simulink model "IC125_K2K_FCB"  (R2018a)
settings: Solver=ode23tb  StartTime=0.0  StopTime=inf  EnableMultiTasking=on
InitFcn:
  | clc
  | init
values from neighbouring files (symbols this model uses):
  C = ( Vout * ( 1 - D ) )/ ( 8 * L * fs^2 * delta_Vout )    (= 0.00125)    [init.m]
  Davis = [6 0.21 0.01453 0].*(404/752.4)    [vehicle_IC125.m]
  gradient_prof_interp_spline_matrix = [0 0.01 0.02 0.03 0.04 0.05 0.06 0.07 0.08 0.09 0.1 0.11 ... (345742 elements, 172871x2)]    [gradient_prof_interp_spline_matrix_kx.mat]    (also in two_way_gradient_interpolated.mat = [1 1.01 1.02 1.03 1.04 1.05 1.06 1.07 1.08 1.09 1.1 1.11 ...)
  inertial_mass = Mass*(1+lambda)    [vehicle_IC125.m]
  L = ( Vout * ( Vin - Vout ) ) / ( Vin * fs * delta_iL )    (= 3.75)    [init.m]
  L_boost = ( Vin_boost * ( Vout_boost - Vin_boost ) ) / ( Vout_boost * delta_iL * fs_boost )    (= 0.0586666666667)    [init.m]
  lambda = 0.08    [vehicle_IC125.m]
  radius = 0.4064    [init.m]
  vel_profile = [0 0.43434 0.4425696 0.4489704 0.4553712 0.461772 0.603504 0.9153144 0.9253728 0.928116 1.0296144 1.0314432 ... (6854 elements, 3427x2)]    [route_KingsX_NewC_KingsX.mat]
undefined symbols (not defined in the file or in its folder): gradient_prof, Ion, Lithium
libraries: powerlib x30, simulink x9, powerlib_meascontrol x5, electricdrivelib x2
settings Model: Creator=hegazi  LastModifiedBy=hegazi
settings SolverCC: ZeroCrossControl=DisableAll  DecoupledContinuousIntegration=on
settings DataIOCC: SaveFormat=Structure  SaveOutput=off  SaveState=on  SignalLogging=off  DSMLogging=off  ReturnWorkspaceOutputs=on  ReturnWorkspaceOutputsName=tp19da9ac7_18bf_45fb_8707_61b44884cc90
settings OptimizationCC: EfficientMapNaN2IntZero=off  LifeSpan=inf
settings DebuggingCC: SFUnexpectedBacktrackingDiag=warning  SFNoUnconditionalDefaultTransitionDiag=warning  SFExecutionAtInitializationDiag=none
settings HardwareCC: ProdBitPerPointer=32  ProdBitPerSizeT=32  ProdBitPerPtrDiffT=32  ProdLargestAtomicFloat=None  ProdIntDivRoundTo=Undefined  ProdEndianess=Unspecified  ProdWordSize=32  ProdHWDeviceType=32-bit Generic  TargetBitPerPointer=64  TargetBitPerSizeT=64  TargetBitPerPtrDiffT=64  TargetLongLongMode=on  TargetIntDivRoundTo=Zero  TargetEndianess=LittleEndian  TargetWordSize=64  TargetHWDeviceType=MATLAB Host  ProdEqTarget=off
settings ModelReferenceCC: PropagateSignalLabelsOutOfModel=off
settings CodeAppCC: MaxIdLength=128
settings GRTTargetCC: TargetLangStandard=C89/C90 (ANSI)  CombineOutputUpdateFcns=off  GRTInterface=on
settings ConfigComp: CovMetricSettings=dw  CovHtmlReporting=on  CovSaveCumulativeToWorkspaceVar=on  CovSaveSingleToWorkspaceVar=on  CovExternalEMLEnable=off
settings SimscapeCC: SimscapeNormalizeSystem=off  SimscapeLogType=all  SimscapeLogSimulationStatistics=on  SimscapeLogLimitData=off

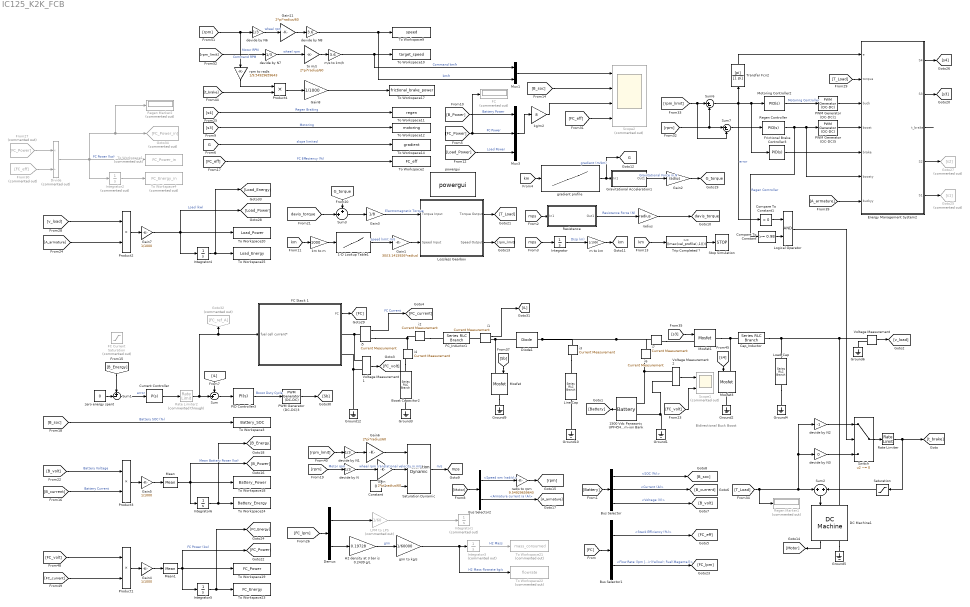
== system IC125_K2K_FCB ==
  note: Bidirectional Buck Boost
  1-D Lookup Table1 : Lookup_n-D  NumberOfTableDimensions=1  BreakpointsForDimension1=vel_profile(:,1)*1000  BreakpointsForDimension2=linspace(min(gradient_prof(:,2)),max(gradient_prof(:,2)),190)  BreakpointsForDimension1DataTypeStr=Inherit: Inherit from 'Breakpoint data'  IndexSearchMethod=Linear search  BeginIndexSearchUsingPreviousIndexResult=on  Table=vel_profile(:,2)*0.277778  TableDataTypeStr=Inherit: Inherit from 'Table data'  InterpMethod=Flat  RemoveProtectionInput=on  InternalRulePriority=Speed  RndMeth=Simplest  SaturateOnIntegerOverflow=on  InputSameDT=on
  1500 Vdc Panasonic UPF454261 Lithium-ion Bank : electricdrivelib/Extra Sources/Battery  BatType=Lithium-Ion  ShowTempParam=off  ThermalPreset=no  ShowAgeParam=off  NomV=3.7*405  NomQ=50  SOC=50  Batt_Tr=30  PresetModel=on  MaxQ=50  MinV=1123.875  FullV=1744.2347  Dis_rate=21.7391  R=0.2997  Normal_OP=45.2174  expZone="[1618.9582      2.4565217]"  current=[1.5 3]  Units=Ampere-hour  Tci=20  NomT=25  T2=0  MaxQ2=2.208  FullV2=3.45  Normal_OP2=2.8  expZone2="[3.22        0.23]"  Rca=0.6  ti=1000  Dp=0  Neq0=0  Tsim=1e6  Ta1=25  Qeol=5.4*0.9  Reol=0.013333*1.2  Char_age=[2.3478, 3]  Dis_age=[2.3478, 10]  N1=1500  N2=10500  N3=1000  N4=1400  Ta2=45  N5=950
  Boost Capacitor2 : powerlib/Elements/Series RLC Branch  LConnTagsString=__new0  RConnTagsString=__new0  BranchType=RC  Resistance=1  Inductance=1e-3  SetiL0=off  InitialCurrent=0  Capacitance=1e-3  Setx0=on  InitialVoltage=400  Measurements=None
  Bus Selector : BusSelector  OutputSignals=SOC (%),Current (A),Voltage (V)
  Bus Selector1 : BusSelector  OutputSignals=Stack Efficiency (%),Flow Rate (lpm [Air(Yellow); Fuel(Magenta)]
  Bus Selector2 : BusSelector  OutputSignals=Speed wm (rad/s),Armature current ia (A)
  Cap_Inductor : powerlib/Elements/Series RLC Branch  LConnTagsString=__new0  RConnTagsString=__new0  BranchType=L  Resistance=1  Inductance=L  SetiL0=off  InitialCurrent=1  Capacitance=1e-6  Setx0=off  InitialVoltage=0  Measurements=Branch voltage and current
  Compare To Constant : simulink/Logic and Bit Operations/Compare To Constant  relop=>=  const=0.98  OutDataTypeStr=boolean
  Compare To Constant1 : simulink/Logic and Bit Operations/Compare To Constant  relop=<  const=0  OutDataTypeStr=boolean
  Constant : Constant  Value=0
  Current Controller : simulink/Continuous/PID Controller  Controller=P  TimeDomain=Continuous-time  SampleTime=-1  IntegratorMethod=Forward Euler  FilterMethod=Forward Euler  Form=Parallel  UseFilter=on  ControllerParametersSource=internal  P=0.5  I=0.001  D=-6.1007201679259e-06  N=246.043739643854  InitialConditionSource=internal  InitialConditionForIntegrator=0  InitialConditionForFilter=0  ExternalReset=none  ZeroCross=off  LimitOutput=off  UpperSaturationLimit=300  LowerSaturationLimit=0  LinearizeAsGain=on  AntiWindupMode=none  Kb=1  TrackingMode=off  Kt=1  PParamMin=[]  PParamMax=[]  IParamMin=[]  IParamMax=[]  DParamMin=[]  DParamMax=[]  NParamMin=[]  NParamMax=[]  KbParamMin=[]  KbParamMax=[]  KtParamMin=[]  KtParamMax=[]  POutMin=[]  POutMax=[]  IOutMin=[]  IOutMax=[]  DOutMin=[]  DOutMax=[]  NOutMin=[]  NOutMax=[]  KbOutMin=[]  KbOutMax=[]  KtOutMin=[]  KtOutMax=[]  IntegratorOutMin=[]  IntegratorOutMax=[]  FilterOutMin=[]  FilterOutMax=[]  SumOutMin=[]  SumOutMax=[]  SumI1OutMin=[]  SumI1OutMax=[]  SumI2OutMin=[]  SumI2OutMax=[]  SumI3OutMin=[]  SumI3OutMax=[]  SumDOutMin=[]  SumDOutMax=[]  SaturationOutMin=[]  SaturationOutMax=[]  IntegratorContinuousStateAttributes=''  IntegratorStateMustResolveToSignalObject=off  IntegratorRTWStateStorageClass=Auto  FilterContinuousStateAttributes=''  FilterStateMustResolveToSignalObject=off  FilterRTWStateStorageClass=Auto  DifferentiatorICPrevScaledInput=0  DifferentiatorOutMin=[]  DifferentiatorOutMax=[]  InitialConditionSetting=State (most efficient)  FilterDiffOutCoefMin=[]  FilterDiffOutCoefMax=[]  SumDenOutMin=[]  SumDenOutMax=[]  SumNumOutMin=[]  SumNumOutMax=[]  ReciprocalOutMin=[]  ReciprocalOutMax=[]  DivideOutMin=[]  DivideOutMax=[]  TunerSelectOption=Transfer Function Based (PID Tuner App)
  DC Machine1 : powerlib/Machines/DC Machine  PresetModel=No  MechanicalLoad=Torque TL  FieldType=Permanent magnet  ShowDetailedParameters=on  MeasurementBus=off  RLa=[0.1499 0.002884]  RLf=[51.14 5.968]  Laf=0.4365  MachineConstant=Torque constant (N.m/A)  Ke=1.8  Kt=1.8  J=0.5106  Bm=0.01383  Tf=13.22  w0=1*(vel_profile(1,2)./(2*pi*radius/60)*3)/9.54929659643  Ifinit=0  TsPowergui=0  TsBlock=-1
  Demux : Demux  Outputs=2
  Diode1 : powerlib/Power Electronics/Diode  Ron=0.001  Lon=0  Vf=0.8  IC=0  UseSnubber=off  Rs=500  Cs=250e-9  Measurements=off
  Divide : Product  Commented=on  Inputs=*/
  Energy Management System2 : State Transition Table  TreatAsAtomicUnit=on
  FC : Display  Commented=on
  FC Current Saturation : Saturate  Commented=on  UpperLimit=50  LowerLimit=0  OutMax=62.5
  FC Stack 1 : Subsystem
      mask Display: image(imread('power_FCV_powertrain_stack.bmp'))
  FC_Inductor1 : powerlib/Elements/Series RLC Branch  LConnTagsString=__new0  RConnTagsString=__new0  BranchType=L  Resistance=0.1  Inductance=L_boost  SetiL0=off  InitialCurrent=1  Capacitance=1e-6  Setx0=off  InitialVoltage=0  Measurements=Branch voltage and current
  Frictional Brake Controller3 : simulink/Continuous/PID Controller  Controller=PID  TimeDomain=Continuous-time  SampleTime=-1  IntegratorMethod=Forward Euler  FilterMethod=Forward Euler  Form=Parallel  UseFilter=on  ControllerParametersSource=internal  P=-0.214642815578935  I=-0.15951379317719  D=-0.00934490052913337  N=15.3222973940802  InitialConditionSource=internal  InitialConditionForIntegrator=0  InitialConditionForFilter=0  ExternalReset=none  LimitOutput=off  UpperSaturationLimit=inf  LowerSaturationLimit=0  LinearizeAsGain=on  AntiWindupMode=none  Kb=1  TrackingMode=off  Kt=1  PParamMin=[]  PParamMax=[]  IParamMin=[]  IParamMax=[]  DParamMin=[]  DParamMax=[]  NParamMin=[]  NParamMax=[]  KbParamMin=[]  KbParamMax=[]  KtParamMin=[]  KtParamMax=[]  POutMin=[]  POutMax=[]  IOutMin=[]  IOutMax=[]  DOutMin=[]  DOutMax=[]  NOutMin=[]  NOutMax=[]  KbOutMin=[]  KbOutMax=[]  KtOutMin=[]  KtOutMax=[]  IntegratorOutMin=[]  IntegratorOutMax=[]  FilterOutMin=[]  FilterOutMax=[]  SumOutMin=[]  SumOutMax=[]  SumI1OutMin=[]  SumI1OutMax=[]  SumI2OutMin=[]  SumI2OutMax=[]  SumI3OutMin=[]  SumI3OutMax=[]  SumDOutMin=[]  SumDOutMax=[]  SaturationOutMin=[]  SaturationOutMax=[]  IntegratorContinuousStateAttributes=''  IntegratorStateMustResolveToSignalObject=off  IntegratorRTWStateStorageClass=Auto  FilterContinuousStateAttributes=''  FilterStateMustResolveToSignalObject=off  FilterRTWStateStorageClass=Auto  DifferentiatorICPrevScaledInput=0  DifferentiatorOutMin=[]  DifferentiatorOutMax=[]  InitialConditionSetting=State (most efficient)  FilterDiffOutCoefMin=[]  FilterDiffOutCoefMax=[]  SumDenOutMin=[]  SumDenOutMax=[]  SumNumOutMin=[]  SumNumOutMax=[]  ReciprocalOutMin=[]  ReciprocalOutMax=[]  DivideOutMin=[]  DivideOutMax=[]  TunerSelectOption=Transfer Function Based (PID Tuner App)
  From27 : From  Commented=on  GotoTag=FC_Power
  From30 : From  Commented=on  GotoTag=FC_eff
  Gain : Gain  Gain=2*pi*radius/60
  Gain1 : Gain  Gain=30/(3.1415926*radius)
  Gain11 : Gain  Gain=2*pi*radius/60
  Gain2 : Gain  Gain=radius
  Gain3 : Gain  Gain=1/8
  Gain{4..5,7..8} (4 alike) : Gain  Gain=1/1000
  Gain6 : Gain  Gain=2*pi*radius/60
  Goto25 : Goto  Commented=on  GotoTag=s1
  Goto27 : Goto  Commented=on  GotoTag=s2
  Goto32 : Goto  Commented=on  GotoTag=FC_ref_A
  Goto34 : Goto  Commented=on  GotoTag=FC_Power_in
  Gravitational Acceleration1 : Subsystem
  Ground{1..6,9..10,12} (9 alike) : powerlib/Elements/Ground  LConnTagsString=a
  H2 density at 3 bar is 0.2439 g/L : Gain  Gain=0.19728
  Integrator : Integrator  InitialCondition=vel_profile(2,1)  ZeroCross=off
  Integrator1 : Integrator  Commented=on  ZeroCross=off
  Integrator2 : Integrator  Commented=on  LimitOutput=on  UpperSaturationLimit=500  LowerSaturationLimit=0  ZeroCross=off
  Integrator3 : Integrator  Commented=on  ZeroCross=off
  Integrator4 : Integrator  ZeroCross=off
  Integrator5 : Integrator  ZeroCross=off
  Integrator6 : Integrator  ZeroCross=off
  LPM to LPS : Gain  Commented=on  Gain=1/60
  Line Cap : powerlib/Elements/Series RLC Branch  LConnTagsString=__new0  RConnTagsString=__new0  BranchType=RC  Resistance=0.0000000000001  Inductance=1e-3  SetiL0=off  InitialCurrent=0  Capacitance=1e-1  Setx0=on  InitialVoltage=1580  Measurements=None
  Load_Cap : powerlib/Elements/Series RLC Branch  LConnTagsString=__new0  RConnTagsString=__new0  BranchType=C  Resistance=1  Inductance=1e-3  SetiL0=off  InitialCurrent=0  Capacitance=C*10  Setx0=off  InitialVoltage=500  Measurements=Branch voltage and current
  Logical Operator : Logic  AllPortsSameDT=off  OutDataTypeStr=boolean
  Lossless Gearbox : Subsystem  mask{N=3}
      mask prompts: N "Gear Ratio"
      mask Display: image(imread('gearbox.jpg'))
  Mean : powerlib_meascontrol/Measurements/Mean  Freq=1  Vinit=0  Ts=0
  Mean1 : powerlib_meascontrol/Measurements/Mean  Freq=1  Vinit=0  Ts=0
  Mosfet : powerlib/Power Electronics/Mosfet  Ron=0.1  Lon=0  Rd=0.01  Vfd=0  IC=0  Rs=1e5  Cs=inf  Measurements=off
  Mosfet1 : powerlib/Power Electronics/Mosfet  Ron=0.1  Lon=0  Rd=0.01  Vfd=0  IC=0  Rs=1e5  Cs=inf  Measurements=off
  Mosfet3 : powerlib/Power Electronics/Mosfet  Ron=0.1  Lon=0  Rd=0.01  Vfd=0  IC=0  Rs=1e5  Cs=inf  Measurements=off
  Motoring Controller2 : simulink/Continuous/PID Controller  Controller=PID  TimeDomain=Continuous-time  SampleTime=-1  IntegratorMethod=Forward Euler  FilterMethod=Forward Euler  Form=Parallel  UseFilter=on  ControllerParametersSource=internal  P=0.0168081368407346  I=0.01166650788265202  D=0.00626354102809722  N=66.8094473612698  InitialConditionSource=internal  InitialConditionForIntegrator=0  InitialConditionForFilter=0  ExternalReset=none  ZeroCross=off  LimitOutput=on  UpperSaturationLimit=1  LowerSaturationLimit=0  LinearizeAsGain=on  AntiWindupMode=none  Kb=1  TrackingMode=off  Kt=1  PParamMin=[]  PParamMax=[]  IParamMin=[]  IParamMax=[]  DParamMin=[]  DParamMax=[]  NParamMin=[]  NParamMax=[]  KbParamMin=[]  KbParamMax=[]  KtParamMin=[]  KtParamMax=[]  POutMin=[]  POutMax=[]  IOutMin=[]  IOutMax=[]  DOutMin=[]  DOutMax=[]  NOutMin=[]  NOutMax=[]  KbOutMin=[]  KbOutMax=[]  KtOutMin=[]  KtOutMax=[]  IntegratorOutMin=[]  IntegratorOutMax=[]  FilterOutMin=[]  FilterOutMax=[]  SumOutMin=[]  SumOutMax=[]  SumI1OutMin=[]  SumI1OutMax=[]  SumI2OutMin=[]  SumI2OutMax=[]  SumI3OutMin=[]  SumI3OutMax=[]  SumDOutMin=[]  SumDOutMax=[]  SaturationOutMin=[]  SaturationOutMax=[]  IntegratorContinuousStateAttributes=''  IntegratorStateMustResolveToSignalObject=off  IntegratorRTWStateStorageClass=Auto  FilterContinuousStateAttributes=''  FilterStateMustResolveToSignalObject=off  FilterRTWStateStorageClass=Auto  DifferentiatorICPrevScaledInput=0  DifferentiatorOutMin=[]  DifferentiatorOutMax=[]  InitialConditionSetting=State (most efficient)  FilterDiffOutCoefMin=[]  FilterDiffOutCoefMax=[]  SumDenOutMin=[]  SumDenOutMax=[]  SumNumOutMin=[]  SumNumOutMax=[]  ReciprocalOutMin=[]  ReciprocalOutMax=[]  DivideOutMin=[]  DivideOutMax=[]  TunerSelectOption=Transfer Function Based (PID Tuner App)
  Mux1 : Mux  Inputs=2
  Mux3 : Mux  Inputs=3
  PID Controller3 : simulink/Continuous/PID Controller  Controller=PI  TimeDomain=Continuous-time  SampleTime=-1  IntegratorMethod=Forward Euler  FilterMethod=Forward Euler  Form=Parallel  UseFilter=on  ControllerParametersSource=internal  P=0.00150104400463717  I=0.095515581062299  D=-6.1007201679259e-06  N=246.043739643854  InitialConditionSource=internal  InitialConditionForIntegrator=0  InitialConditionForFilter=0  ExternalReset=none  ZeroCross=off  LimitOutput=on  UpperSaturationLimit=1  LowerSaturationLimit=0  LinearizeAsGain=on  AntiWindupMode=none  Kb=1  TrackingMode=off  Kt=1  PParamMin=[]  PParamMax=[]  IParamMin=[]  IParamMax=[]  DParamMin=[]  DParamMax=[]  NParamMin=[]  NParamMax=[]  KbParamMin=[]  KbParamMax=[]  KtParamMin=[]  KtParamMax=[]  POutMin=[]  POutMax=[]  IOutMin=[]  IOutMax=[]  DOutMin=[]  DOutMax=[]  NOutMin=[]  NOutMax=[]  KbOutMin=[]  KbOutMax=[]  KtOutMin=[]  KtOutMax=[]  IntegratorOutMin=[]  IntegratorOutMax=[]  FilterOutMin=[]  FilterOutMax=[]  SumOutMin=[]  SumOutMax=[]  SumI1OutMin=[]  SumI1OutMax=[]  SumI2OutMin=[]  SumI2OutMax=[]  SumI3OutMin=[]  SumI3OutMax=[]  SumDOutMin=[]  SumDOutMax=[]  SaturationOutMin=[]  SaturationOutMax=[]  IntegratorContinuousStateAttributes=''  IntegratorStateMustResolveToSignalObject=off  IntegratorRTWStateStorageClass=Auto  FilterContinuousStateAttributes=''  FilterStateMustResolveToSignalObject=off  FilterRTWStateStorageClass=Auto  DifferentiatorICPrevScaledInput=0  DifferentiatorOutMin=[]  DifferentiatorOutMax=[]  InitialConditionSetting=State (most efficient)  FilterDiffOutCoefMin=[]  FilterDiffOutCoefMax=[]  SumDenOutMin=[]  SumDenOutMax=[]  SumNumOutMin=[]  SumNumOutMax=[]  ReciprocalOutMin=[]  ReciprocalOutMax=[]  DivideOutMin=[]  DivideOutMax=[]  TunerSelectOption=Transfer Function Based (PID Tuner App)
  PWM Generator (DC-DC)1 : powerlib_meascontrol/Pulse & Signal Generators/PWM Generator (DC-DC)  Fsw=350  Ts=0
  PWM Generator (DC-DC)3 : powerlib_meascontrol/Pulse & Signal Generators/PWM Generator (DC-DC)  Fsw=500  Ts=0
  PWM Generator (DC-DC)5 : powerlib_meascontrol/Pulse & Signal Generators/PWM Generator (DC-DC)  Fsw=350  Ts=0
  Product{1..4} (4 alike) : Product
  Rate Limiter : RateLimiter  RisingSlewLimit=1000  FallingSlewLimit=-1000  SampleTimeMode=inherited
  Rate Limiter2 : RateLimiter  Commented=through  RisingSlewLimit=100  FallingSlewLimit=-100  SampleTimeMode=inherited
  Regen Controller : simulink/Continuous/PID Controller  Controller=PID  TimeDomain=Continuous-time  SampleTime=-1  IntegratorMethod=Forward Euler  FilterMethod=Forward Euler  Form=Parallel  UseFilter=on  ControllerParametersSource=internal  P=0.0168081368407346  I=0.01166650788265202  D=0.00626354102809722  N=66.8094473612698  InitialConditionSource=internal  InitialConditionForIntegrator=0  InitialConditionForFilter=0  ExternalReset=none  ZeroCross=off  LimitOutput=on  UpperSaturationLimit=1  LowerSaturationLimit=0  LinearizeAsGain=on  AntiWindupMode=none  Kb=1  TrackingMode=off  Kt=1  PParamMin=[]  PParamMax=[]  IParamMin=[]  IParamMax=[]  DParamMin=[]  DParamMax=[]  NParamMin=[]  NParamMax=[]  KbParamMin=[]  KbParamMax=[]  KtParamMin=[]  KtParamMax=[]  POutMin=[]  POutMax=[]  IOutMin=[]  IOutMax=[]  DOutMin=[]  DOutMax=[]  NOutMin=[]  NOutMax=[]  KbOutMin=[]  KbOutMax=[]  KtOutMin=[]  KtOutMax=[]  IntegratorOutMin=[]  IntegratorOutMax=[]  FilterOutMin=[]  FilterOutMax=[]  SumOutMin=[]  SumOutMax=[]  SumI1OutMin=[]  SumI1OutMax=[]  SumI2OutMin=[]  SumI2OutMax=[]  SumI3OutMin=[]  SumI3OutMax=[]  SumDOutMin=[]  SumDOutMax=[]  SaturationOutMin=[]  SaturationOutMax=[]  IntegratorContinuousStateAttributes=''  IntegratorStateMustResolveToSignalObject=off  IntegratorRTWStateStorageClass=Auto  FilterContinuousStateAttributes=''  FilterStateMustResolveToSignalObject=off  FilterRTWStateStorageClass=Auto  DifferentiatorICPrevScaledInput=0  DifferentiatorOutMin=[]  DifferentiatorOutMax=[]  InitialConditionSetting=State (most efficient)  FilterDiffOutCoefMin=[]  FilterDiffOutCoefMax=[]  SumDenOutMin=[]  SumDenOutMax=[]  SumNumOutMin=[]  SumNumOutMax=[]  ReciprocalOutMin=[]  ReciprocalOutMax=[]  DivideOutMin=[]  DivideOutMax=[]  TunerSelectOption=Transfer Function Based (PID Tuner App)
  Regen Marker1 : Display  Commented=on
  Regen Marker2 : Display  Commented=on
  Resistance : Subsystem
  Saturation : Saturate  UpperLimit=inf  LowerLimit=0
  Saturation Dynamic : simulink/Discontinuities/Saturation Dynamic  OutMin=[]  OutMax=[]  OutDataTypeStr=Inherit: Same as second input  OutDataType=fixdt(1, 16)  OutScaling=2^-10  DoSatur=off
  Scope1 : Scope  Commented=on  NumInputPorts=2
  Scope2 : Scope  Commented=on  NumInputPorts=4
  Stop Simulation : Stop
  Sum : Sum  Inputs=-+|
  Sum1 : Sum  Inputs=+-|
  Sum2 : Sum  Inputs=+|+
  Sum3 : Sum  Inputs=++|
  Sum6 : Sum  Inputs=|+-
  Sum7 : Sum  Inputs=|+-
  Switch : Switch  Criteria=u2 ~= 0
  To Workspace1 : ToWorkspace  Commented=on  VariableName=FC_Power_in  SaveFormat=Timeseries  SampleTime=1
  To Workspace10 : ToWorkspace  VariableName=target_speed  SaveFormat=Timeseries  SampleTime=1
  To Workspace11 : ToWorkspace  VariableName=regen  SaveFormat=Timeseries  SampleTime=1
  To Workspace12 : ToWorkspace  VariableName=motoring  SaveFormat=Timeseries  SampleTime=1
  To Workspace14 : ToWorkspace  VariableName=gradient  SaveFormat=Timeseries  SampleTime=1
  To Workspace17 : ToWorkspace  VariableName=frictional_brake_power  SaveFormat=Timeseries  SampleTime=1
  To Workspace18 : ToWorkspace  VariableName=Battery_Power  SaveFormat=Timeseries  SampleTime=1
  To Workspace19 : ToWorkspace  VariableName=FC_Power  SaveFormat=Timeseries  SampleTime=1
  To Workspace2 : ToWorkspace  VariableName=FC_eff  SaveFormat=Timeseries  SampleTime=1
  To Workspace20 : ToWorkspace  VariableName=Load_Power  SaveFormat=Timeseries  SampleTime=1
  To Workspace21 : ToWorkspace  Commented=on  VariableName=mass_consumed  SaveFormat=Timeseries  SampleTime=1
  To Workspace22 : ToWorkspace  Commented=on  VariableName=flowrate  SaveFormat=Timeseries  SampleTime=1
  To Workspace23 : ToWorkspace  VariableName=FC_Energy  SaveFormat=Timeseries  SampleTime=1
  To Workspace24 : ToWorkspace  VariableName=Battery_Energy  SaveFormat=Timeseries  SampleTime=1
  To Workspace25 : ToWorkspace  VariableName=Load_Energy  SaveFormat=Timeseries  SampleTime=1
  To Workspace3 : ToWorkspace  VariableName=Battery_SOC  SaveFormat=Timeseries  SampleTime=1
  To Workspace4 : ToWorkspace  Commented=on  VariableName=FC_Energy_in  SaveFormat=Timeseries  SampleTime=1
  To Workspace9 : ToWorkspace  VariableName=speed  SaveFormat=Timeseries  SampleTime=1
  Transfer Fcn2 : TransferFcn  Numerator=[pi]  Denominator=[1 pi]
  Trip Completed ? : simulink/Logic and Bit Operations/Compare To Constant  relop=>=  const=((max(vel_profile(:,1))))  OutDataTypeStr=boolean
  Voltage Measurement : powerlib/Measurements/Voltage Measurement  PhasorSimulation=off  OutputType=Complex  PSBequivalent=0
  Voltage Measurement1 : powerlib/Measurements/Voltage Measurement  PhasorSimulation=off  OutputType=Complex  PSBequivalent=0
  Voltage Measurement2 : powerlib/Measurements/Voltage Measurement  PhasorSimulation=off  OutputType=Complex  PSBequivalent=0
  devide by N{,1,6..7} (4 alike) : Gain  Gain=1/3
  devide by N2 : Gain  Gain=-1
  devide by N3 : Gain  Gain=0
  devide by N8 : Gain  Gain=3.6
  g/m to kg/s : Gain  Gain=1/60000
  gradient profile : Lookup_n-D  NumberOfTableDimensions=1  BreakpointsForDimension1=gradient_prof_interp_spline_matrix(:,1)  BreakpointsForDimension2=linspace(min(gradient_prof(:,2)),max(gradient_prof(:,2)),190)  BreakpointsForDimension1DataTypeStr=Inherit: Inherit from 'Breakpoint data'  IndexSearchMethod=Linear search  Table=gradient_prof_interp_spline_matrix(:,2)  TableDataTypeStr=Inherit: Inherit from 'Table data'  ExtrapMethod=Clip  RemoveProtectionInput=on  InternalRulePriority=Speed  RndMeth=Simplest  SaturateOnIntegerOverflow=on  InputSameDT=on
  i{1..7} (7 alike) : powerlib/Measurements/Current Measurement  PhasorSimulation=off  OutputType=Complex  PSBequivalent=0
  kg/m2 : Gain  Gain=8
  km to m : Gain  Gain=1000
  m to km : Gain  Gain=1/1000
  m/s to km/h : Gain  Gain=3.6
  powergui : powerlib/powergui  Priority=1  SimulationMode=Continuous  SampleTime=1e-5  frequency=60  Iterations=50  frequencyindice=0  Pbase=100e6  ErrMax=1e-4  UnitsV=kV  UnitsW=MW  buscounter=0  FunctionMessages=off  echomessages=off  EnableUseOfTLC=off  CurrentSourceSwitches=off  DisableSnubberDevices=on  DisableRonSwitches=on  DisableVfSwitches=on  DisplayEquations=off  SolverType=Tustin  Interpol=off  ExternalGateDelay=off  methode=off  Ts=0  x0status=blocks  SPID=on  SwTol=0  HookPort=off  RestoreLinks=warning  ResistiveCurrentMeasurement=off  Frange=[0:2:500]  Ylog=off  Xlog=on  ShowGrid=off  save=off  variable=ZData  structure=0  ZoomFFT=off  StartTime=0.0  cycles=1  DisplayStyle=1  fundamental=60  FreqAxis=off  MaxFrequency=1000  frequencyindicesteady=1  RmsSteady=1  display=off
  rad/s to rpm : Gain  Gain=9.54929659643
  radius : Gain  Gain=radius
  rpm to rad/s : Gain  Gain=1/9.54929659643
  to m/s : Gain  Gain=2*pi*radius/60
  zero energy spent : Constant  Value=0
  tag scope: G=global, G_torque=global, davis_torque=global, km=global, mps=global
  wires:
  DC Machine1/1 -> [Motor]
  Voltage Measurement/1 -> [v_load]
  Trip Completed ?/1 -> Stop Simulation/1
  [rpm] -> devide by N/1  "Motor rpm"
  Gain3/1 -> Lossless Gearbox/1(Torque Input)  "Electromagnetic Torque"
  Lossless Gearbox/2(Speed Output) -> [rpm_limit]
  Lossless Gearbox/1(Torque Output) -> [T_Load]
  devide by N/1 -> Gain/1  "wheel rpm"
  Gain/1 -> Saturation Dynamic/2  "translational velocity in m/s"
  [davis_torque] -> Sum3/2
  Sum3/1 -> Gain3/1
  Constant/1 -> Saturation Dynamic/3
  [rpm_limit] -> devide by N1/1
  devide by N1/1 -> Gain6/1
  Sum2/1 -> DC Machine1/1
  Gain6/1 -> Saturation Dynamic/1
  1500 Vdc Panasonic UPF454261 Lithium-ion Bank/1 -> [Battery]
  [s4] -> Mosfet3/1
  [FC] -> Bus Selector1/1
  [Battery] -> Bus Selector/1
  Bus Selector1/1 -> [FC_eff]  "<Stack Efficiency (%)>"
  [Motor] -> Bus Selector2/1
  Bus Selector2/2 -> [A_armature]  "<Armature current ia (A)>"
  Bus Selector2/1 -> rad/s to rpm/1  "<Speed wm (rad/s)>"
  rad/s to rpm/1 -> [rpm]
  Bus Selector1/2 -> [FC_lpm]  "<Flow Rate (lpm [Air(Yellow); Fuel(Magenta)]>"
  [T_Load] -> Regen Marker1/1, Sum2/1, devide by N3/1, devide by N2/1
  Saturation Dynamic/1 -> [mps]  "m/s"
  Resistance/1(Out1) -> radius/1  "Resistance Force (N)"
  radius/1 -> [davis_torque]
  [mps] -> Resistance/1(In1)
  Integrator/1 -> m to km/1  "Disp (m)"
  [mps] -> Integrator/1
  m to km/1 -> [km]
  Gravitational Acceleration1/1(Out1) -> Gain2/1  "Gravitational Force in N"
  gradient profile/1 -> Gravitational Acceleration1/1(In1), [G]  "gradient (m/km)"
  [km] -> gradient profile/1
  Gain2/1 -> [G_torque]
  [km] -> km to m/1
  1-D Lookup Table1/1 -> Gain1/1  "speed limit m/s"
  km to m/1 -> 1-D Lookup Table1/1
  [km] -> Trip Completed ?/1
  [G_torque] -> Sum3/1
  Gain1/1 -> Lossless Gearbox/2(Speed Input)
  Bus Selector/2 -> [B_current]  "<Current (A)>"
  Bus Selector/3 -> [B_volt]  "<Voltage (V)>"
  Bus Selector/1 -> [B_soc]  "<SOC (%)>"
  LPM to LPS/1 -> Integrator1/1
  [FC_lpm] -> Demux/1
  Demux/1 -> LPM to LPS/1
  Demux/2 -> H2 density at 3 bar is 0.2439 g/L/1
  FC Stack 1/1(FC) -> [FC]
  Sum/1 -> PID Controller3/1
  PWM Generator (DC-DC)3/1 -> [Sb]
  i1/1 -> [iL]
  [iL] -> Sum/1
  [Sb] -> Mosfet/1
  Sum1/1 -> Current Controller/1  "error"
  [B_Energy] -> Sum1/1
  zero energy spent/1 -> Sum1/2
  Voltage Measurement1/1 -> [FC_volt]
  i5/1 -> [FC_current]  "FC Current"
  [FC_eff] -> To Workspace2/1  "FC Effeciency (%)"
  [FC_current] -> Product1/2
  [FC_volt] -> Product1/1
  [B_current] -> Product3/2  "Battery Current"
  [B_volt] -> Product3/1  "Battery Voltage"
  [A_armature] -> Product2/2
  [v_load] -> Product2/1
  devide by N6/1 -> Gain11/1  "wheel rpm"
  [rpm] -> devide by N6/1, rpm to rad/s/1  "Motor RPM"
  Gain11/1 -> devide by N8/1
  devide by N7/1 -> to m/s/1  "wheel rpm"
  to m/s/1 -> m/s to km/h/1
  [rpm_limit] -> devide by N7/1  "Command RPM"
  devide by N8/1 -> To Workspace9/1, Mux1/2  "km/h"
  m/s to km/h/1 -> To Workspace10/1, Mux1/1  "Command km/h"
  [s4] -> To Workspace11/1  "Regen Braking"
  [s3] -> To Workspace12/1  "Motoring"
  [G] -> To Workspace14/1  "slope limited"
  [rpm] -> Sum7/1, Sum6/2
  Sum7/1 -> Regen Controller/1
  Energy Management System2/4(S2) -> Goto27/1
  Energy Management System2/5(S1) -> Goto25/1
  [rpm_limit] -> Sum6/1, Sum7/2
  Energy Management System2/1(S4) -> [s4]
  Energy Management System2/2(S3) -> [s3]
  [T_Load] -> Energy Management System2/2(torque)
  Energy Management System2/3(t_brake) -> ?
  [A_armature] -> Energy Management System2/7(buckyy)
  Transfer Fcn2/1 -> Energy Management System2/1(e)
  Motoring Controller2/1 -> PWM Generator (DC-DC)1/1  "Motoring Controller"
  Regen Controller/1 -> Energy Management System2/6(boosty), PWM Generator (DC-DC)5/1, Compare To Constant/1  "Regen Controller"
  Sum6/1 -> Frictional Brake Controller3/1, Motoring Controller2/1, Transfer Fcn2/1, Compare To Constant1/1  "error"
  Frictional Brake Controller3/1 -> Energy Management System2/5(brake)
  PWM Generator (DC-DC)1/1 -> Energy Management System2/3(buck)
  Product2/1 -> Gain7/1
  Product1/1 -> Gain4/1
  Product3/1 -> Gain5/1
  Gain4/1 -> Mean1/1
  Gain5/1 -> Mean/1
  Gain7/1 -> [Load_Power], Integrator4/1, To Workspace20/1  "Load (kw)"
  Mux3/1 -> kg/m2/1
  Mux1/1 -> Scope2/1
  PWM Generator (DC-DC)5/1 -> Energy Management System2/4(boost)
  [s3] -> Mosfet1/1
  Switch/1 -> Rate Limiter/1
  Compare To Constant/1 -> Logical Operator/2
  Logical Operator/1 -> Switch/2
  Compare To Constant1/1 -> Logical Operator/1
  devide by N2/1 -> Switch/1
  devide by N3/1 -> Switch/3
  Rate Limiter/1 -> [t_brake], Saturation/1
  [t_brake] -> Product4/2
  Product4/1 -> Gain8/1
  Gain8/1 -> To Workspace17/1
  rpm to rad/s/1 -> Product4/1
  Saturation/1 -> Sum2/2
  PID Controller3/1 -> PWM Generator (DC-DC)3/1  "Boost Duty Cycle"
  Current Controller/1 -> Rate Limiter2/1
  Mean/1 -> [B_Power], Integrator6/1, To Workspace18/1  "Mean Battery Power (kw)"
  Mean1/1 -> [FC_Power], Integrator5/1, To Workspace19/1  "FC Power (kw)"
  H2 density at 3 bar is 0.2439 g/L/1 -> g/m to kg/s/1  "g/m"
  Integrator3/1 -> To Workspace21/1  "H2 Mass"
  g/m to kg/s/1 -> To Workspace22/1, Integrator3/1  "H2 Mass flowrate kg/s"
  Integrator6/1 -> [B_Energy], To Workspace24/1
  Integrator5/1 -> [FC_Energy], To Workspace23/1
  Integrator4/1 -> [Load_Energy], To Workspace25/1
  [B_soc] -> To Workspace3/1  "Battery SOC (%)"
  [FC_Power] -> FC/1, Mux3/2  "FC Power"
  [B_Power] -> Mux3/1  "Battery Power"
  kg/m2/1 -> Scope2/3
  [Load_Power] -> Mux3/3  "Load Power"
  [B_soc] -> Scope2/2
  [FC_eff] -> Scope2/4
  Rate Limiter2/1 -> Sum/2, FC Stack 1/1(fuel cell current*), Goto32/1
  From30/1 -> Divide/2
  From27/1 -> Divide/1
  Divide/1 -> Regen Marker2/1, Goto34/1, Integrator2/1, To Workspace1/1  "FC Power (kw)"
  Integrator2/1 -> To Workspace4/1
  Voltage Measurement2/1 -> Scope1/1
  [FC_volt] -> Scope1/2
  connections:
  Mosfet1/RConn1 -- Cap_Inductor/LConn1 -- Mosfet3/LConn1
  i4/LConn1 -- i5/RConn1 -- i2/LConn1
  Mosfet/LConn1 -- Diode1/LConn1 -- i1/RConn1
  Voltage Measurement1/LConn2 -- Ground12/LConn1 -- FC Stack 1/RConn2
  i5/LConn1 -- FC Stack 1/RConn1 -- Voltage Measurement1/LConn1
  Cap_Inductor/RConn1 -- Load_Cap/LConn1 -- Voltage Measurement/LConn1 -- DC Machine1/LConn1
  DC Machine1/RConn1 -- Ground5/LConn1
  i7/RConn1 -- Mosfet1/LConn1
  Ground6/LConn1 -- Voltage Measurement/LConn2
  Mosfet/RConn1 -- Ground9/LConn1
  Ground1/LConn1 -- Voltage Measurement2/LConn2 -- 1500 Vdc Panasonic UPF454261 Lithium-ion Bank/LConn2
  Ground10/LConn1 -- Line Cap/RConn1
  i6/RConn1 -- Voltage Measurement2/LConn1 -- 1500 Vdc Panasonic UPF454261 Lithium-ion Bank/LConn1
  Load_Cap/RConn1 -- Ground4/LConn1
  i4/RConn1 -- Boost Capacitor2/LConn1
  i3/RConn1 -- Line Cap/LConn1
  Ground2/LConn1 -- Mosfet3/RConn1
  Ground3/LConn1 -- Boost Capacitor2/RConn1
  i2/RConn1 -- FC_Inductor1/LConn1
  i1/LConn1 -- FC_Inductor1/RConn1
  Diode1/RConn1 -- i7/LConn1 -- i6/LConn1 -- i3/LConn1

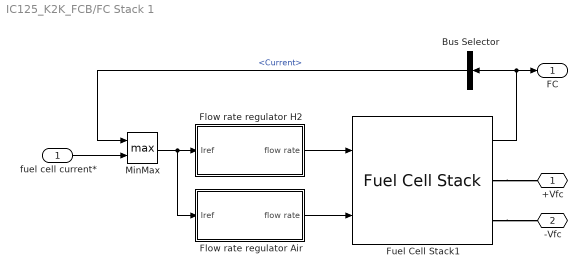
== system IC125_K2K_FCB/FC Stack 1 ==
  fuel cell current* : Inport
  Bus Selector : BusSelector  OutputSignals=Current
  Flow rate regulator Air : Subsystem
  Flow rate regulator H2 : Subsystem
  Fuel Cell Stack1 : electricdrivelib/Extra Sources/Fuel Cell Stack  PresetModel=No (User-Defined)  FcType=Proton Exchange Membrane (PEM)  Detailed=Detailed  Eoc="[400  380]"  NomVI="[285  300]"  EndVI="[347.3           288]"  Nc=400  n=57  TOp=95  AirFr=1698  SuppPress="[3  3]"  Comp="[99.95           21            1]"  SignX=off  SignY=off  FlowRateH2=on  FlowRateAir=on  SystemTemp=off  SystemPH2=off  SystemPAir=off  FCDyn=on  FC_tau=2  Peak_O2=80  V_Under=10
      settings: SourceProductName=Simscape Power Systems  SourceProductBaseCode=PS
  MinMax : MinMax  Function=max  Inputs=2
  +Vfc : PMIOPort  Side=Right
  -Vfc : PMIOPort  Port=2  Side=Right
  FC : Outport
  wires:
  Flow rate regulator H2/1(flow rate) -> Fuel Cell Stack1/1
  Flow rate regulator Air/1(flow rate) -> Fuel Cell Stack1/2
  Bus Selector/1 -> MinMax/1  "<Current>"
  Fuel Cell Stack1/1 -> FC/1, Bus Selector/1
  MinMax/1 -> Flow rate regulator Air/1(Iref), Flow rate regulator H2/1(Iref)
  fuel cell current*/1 -> MinMax/2
  connections:
  Fuel Cell Stack1/RConn2 -- -Vfc/RConn1
  Fuel Cell Stack1/RConn1 -- +Vfc/RConn1

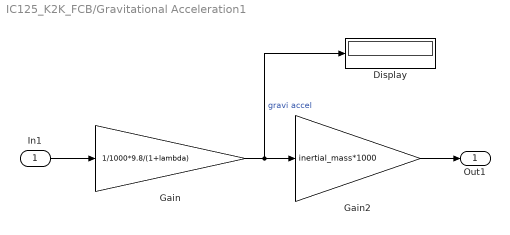
== system IC125_K2K_FCB/Gravitational Acceleration1 ==
  In1 : Inport
  Display : Display
  Gain : Gain  Gain=1/1000*9.8/(1+lambda)
  Gain2 : Gain  Gain=inertial_mass*1000
  Out1 : Outport
  wires:
  Gain/1 -> Gain2/1, Display/1  "gravi accel"
  In1/1 -> Gain/1
  Gain2/1 -> Out1/1

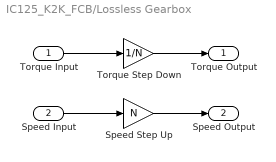
== system IC125_K2K_FCB/Lossless Gearbox ==
  Torque Input : Inport
  Speed Input : Inport  Port=2
  Speed Step Up : Gain  Gain=N
  Torque Step Down : Gain  Gain=1/N
  Torque Output : Outport
  Speed Output : Outport  Port=2
  wires:
  Torque Step Down/1 -> Torque Output/1
  Torque Input/1 -> Torque Step Down/1
  Speed Step Up/1 -> Speed Output/1
  Speed Input/1 -> Speed Step Up/1

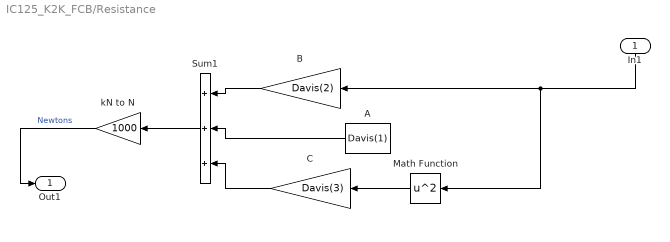
== system IC125_K2K_FCB/Resistance ==
  In1 : Inport
  A : Constant  Value=Davis(1)
  B : Gain  Gain=Davis(2)
  C : Gain  Gain=Davis(3)
  Math Function : Math  Operator=square  SaturateOnIntegerOverflow=on
  Sum1 : Sum  Inputs=+++
  kN to N : Gain  Gain=1000
  Out1 : Outport
  wires:
  Math Function/1 -> C/1
  C/1 -> Sum1/3
  kN to N/1 -> Out1/1  "Newtons"
  Sum1/1 -> kN to N/1
  A/1 -> Sum1/2
  B/1 -> Sum1/1
  In1/1 -> B/1, Math Function/1

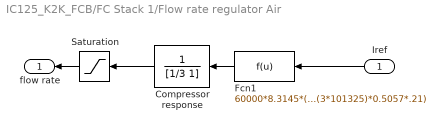
== system IC125_K2K_FCB/FC Stack 1/Flow rate regulator Air ==
  Iref : Inport
  Compressor response : TransferFcn  Denominator=[1/3 1]
  Fcn1 : Fcn  Expr=60000*8.3145*(273+95)*400*u(1)/(4*96485*(3*101325)*0.5057*.21)
  Saturation : Saturate  UpperLimit=inf  LowerLimit=60
  flow rate : Outport
  wires:
  Compressor response/1 -> Saturation/1
  Fcn1/1 -> Compressor response/1
  Saturation/1 -> flow rate/1
  Iref/1 -> Fcn1/1

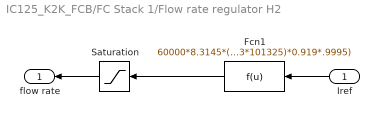
== system IC125_K2K_FCB/FC Stack 1/Flow rate regulator H2 ==
  Iref : Inport
  Fcn1 : Fcn  Expr=60000*8.3145*(273+95)*400*u(1)/(2*96485*(3*101325)*0.919*.9995)
  Saturation : Saturate  UpperLimit=inf  LowerLimit=1
  flow rate : Outport
  wires:
  Iref/1 -> Fcn1/1
  Saturation/1 -> flow rate/1
  Fcn1/1 -> Saturation/1

== stateflow chart IC125_K2K_FCB/Energy Management System2 ==
  state Motoring
    entry:
    S4=0;
    S2=0;
    t_brake=0;
    during:
    S3=buck;
    S1=buck;
  state Regen_Braking
    entry:
    S3=0;
    S1=0;
    t_brake=0;
    during:
    S4=boost;
    S2=boost;
  (default) -> Motoring
  Motoring -> Regen_Braking : [  e < -1 &&  buckyy <= 0 ]
      |
      | % after(1,sec) && boosty ~= 0 &&
  Regen_Braking -> Motoring : [ e > 1 && buckyy > 0]
      |
      | % after(1,sec) &&
  data: e input; torque input; buck input; boost input; S4 output; S3 output; brake input; t_brake output; S2 output; S1 output; boosty input; buckyy input
